simulink model "nivel_tranque_agua"  (R2025a)
settings: Solver=VariableStepAuto  StartTime=0.0  StopTime=20  RelTol=1e-3
libraries: fuzblock x1
settings Model: Creator=Bremdow  LastModifiedBy=Bremdows
settings DebuggingCC: UnconnectedInputMsg=warning  UnconnectedOutputMsg=warning  UnconnectedLineMsg=warning
settings ModelReferenceCC: EnableRefExpFcnMdlSchedulingChecks=on
settings RTWCC: GPUComputeCapability=3.5  DLArmComputeVersion=19.05

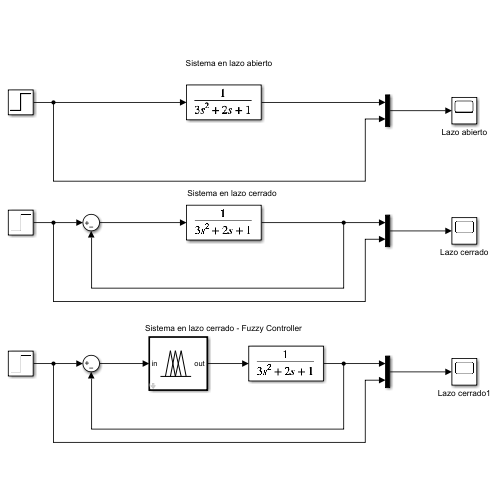
[thumbnail: Simulink's stored preview of the top-level diagram]
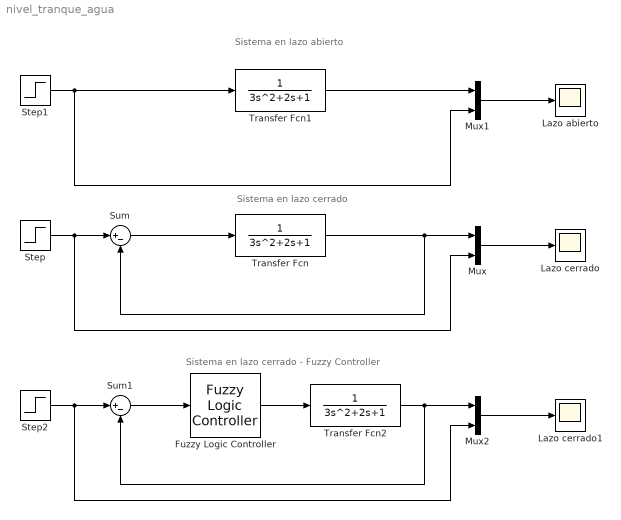
== system nivel_tranque_agua ==
  note: Sistema en lazo cerrado
  note: Sistema en lazo abierto
  note: Sistema en lazo cerrado - Fuzzy Controller
  Fuzzy Logic Controller : fuzblock/Fuzzy Logic  Controller  FIS='tipper.fis'  OutputSampleNumber=101  DataType=double  UseLookupTable=off  NumBreakpoints=10  FuzzifiedInputs=off  RuleFiringStrengths=off  RuleOutputs=off  AggregatedOutputs=off  SimulateUsing=Interpreted execution  OutOfRangeInputValueMessage=warning  NoRuleFiredMessage=warning  EmptyOutputFuzzySetMessage=warning
  Lazo abierto : Scope
      settings: ActiveDisplayYMinimum=-0.1352590605125199  ActiveDisplayYMaximum=1.2499386030113431
  Lazo cerrado : Scope
      settings: ActiveDisplayYMinimum=-1  ActiveDisplayYMaximum=1
  Lazo cerrado1 : Scope
      settings: ActiveDisplayYMinimum=-1  ActiveDisplayYMaximum=1  DataLoggingVariableName=ScopeData2
  Mux : Mux  Inputs=2
  Mux1 : Mux  Inputs=2
  Mux2 : Mux  Inputs=2
  Step : Step  Time=0  SampleTime=0
  Step1 : Step  Time=0  SampleTime=0
  Step2 : Step  Time=0  SampleTime=0
  Sum : Sum  Inputs=|+-
  Sum1 : Sum  Inputs=|+-
  Transfer Fcn : TransferFcn  Denominator=[3 2 1]
  Transfer Fcn1 : TransferFcn  Denominator=[3 2 1]
  Transfer Fcn2 : TransferFcn  Denominator=[3 2 1]
  wires:
  Step/1 -> Mux/2, Sum/1
  Sum/1 -> Transfer Fcn/1
  Transfer Fcn/1 -> Sum/2, Mux/1
  Mux/1 -> Lazo cerrado/1
  Step1/1 -> Transfer Fcn1/1, Mux1/2
  Transfer Fcn1/1 -> Mux1/1
  Mux1/1 -> Lazo abierto/1
  Mux2/1 -> Lazo cerrado1/1
  Transfer Fcn2/1 -> Mux2/1, Sum1/2
  Step2/1 -> Sum1/1, Mux2/2
  Fuzzy Logic Controller/1 -> Transfer Fcn2/1
  Sum1/1 -> Fuzzy Logic Controller/1
